simulink model "PMSM_traditional"  (R2014b)
settings: Solver=ode3  StartTime=0.0  StopTime=0.4  FixedStep=10e-6  RelTol=1e-4
libraries: powerlib x6, simulink x1
settings Model: Creator=ZhuJ  LastModifiedBy=Lei
settings SolverCC: SolverResetMethod=Robust
settings DataIOCC: SignalLoggingSaveFormat=ModelDataLogs
settings OptimizationCC: ExpressionDepthLimit=2147483647  InitFltsAndDblsToZero=on
settings DebuggingCC: UnderspecifiedInitializationDetection=Classic  MergeDetectMultiDrivingBlocksExec=none  FcnCallInpInsideContextMsg=UseLocalSettings  StateNameClashWarn=warning
settings GRTTargetCC: CombineOutputUpdateFcns=off  GRTInterface=on

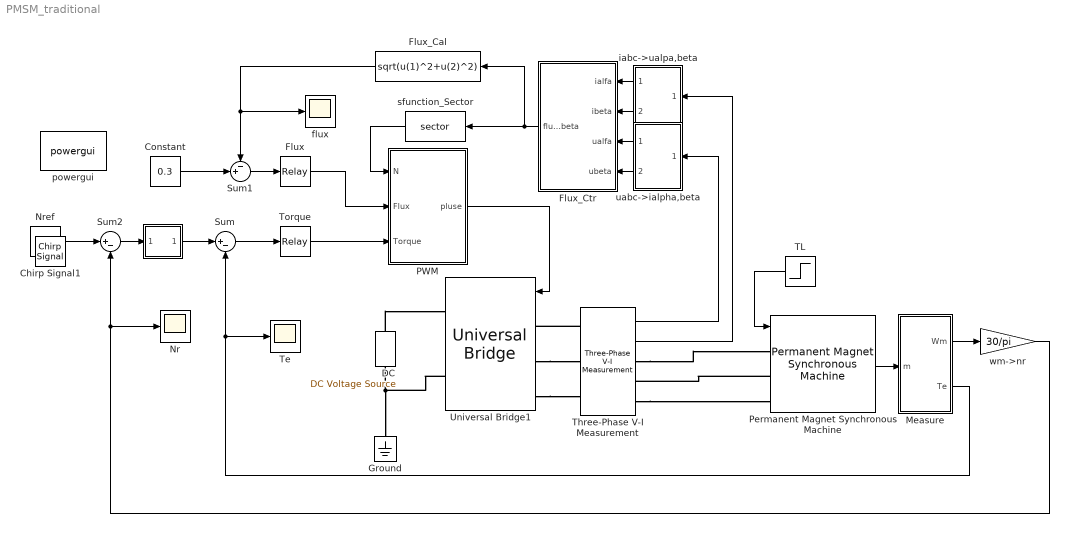
== system PMSM_traditional ==
  "\t" : Subsystem
      mask Display: disp('PI')
  Constant : Constant  Value=0.3
  DC : powerlib/Electrical Sources/DC Voltage Source  Amplitude=311  Measurements=None
  Flux : Relay  OnSwitchValue=0.002  OffSwitchValue=-0.002
  Flux_Cal : Fcn  Expr=sqrt(u(1)^2+u(2)^2)
  Flux_Ctr : Subsystem
  Ground : powerlib/Elements/Ground  LConnTagsString=a
  Measure : Subsystem
  Nr : Scope
      settings: TimeRange=0.3  YMin=595  YMax=620  SaveName=wm  SampleInput=on
  Nref : Constant  Value=600
  PWM : Subsystem
  Permanent Magnet Synchronous Machine : powerlib/Machines/Permanent Magnet Synchronous Machine  NbPhases=3  FluxDistribution=Sinusoidal  RotorType=Salient-pole  MechanicalLoad=Torque Tm  PresetModel=No  ShowDetailedParameters=on  MeasurementBus=off  Resistance=1.2  Inductance=8.5e-3  dqInductances=[8.5e-3,8.5e-3]  La=0.000835  MachineConstant=Flux linkage established by magnets (V.s)  Flux=0.175  VoltageCst=126.966  TorqueCst=1.05  Flat=120  Mechanical=[0.0008 0 4]  PolePairs=4  InitialConditions=[0,0, 0,0]  InitialConditions5ph=[0 0 0 0 0 0]  TsPowergui=0  TsBlock=-1  RefAngle=Aligned with phase A axis (original Park)
  Sum : Sum  Inputs=|+-
  Sum1 : Sum  Inputs=-+|
  Sum2 : Sum  Inputs=|+-
  TL : Step  Time=0.2  After=1.5  SampleTime=0
  Te : Scope
      settings: YMin=-2  SaveName=Te  SampleInput=on
  Three-Phase V-I Measurement : powerlib/Measurements/Three-Phase V-I Measurement  VoltageMeasurement=phase-to-ground  SetLabelV=off  LabelV=Vabc  Vpu=off  VpuLL=off  CurrentMeasurement=yes  SetLabelI=off  LabelI=Iabc  Ipu=off  Pbase=100e6  Vbase=500e3  OutputType=Complex  PhasorSimulation=off  PSBequivalent=0
  Torque : Relay  OnSwitchValue=0.1  OffSwitchValue=-0.1
  Universal Bridge1 : powerlib/Power Electronics/Universal Bridge  Arms=3  SnubberResistance=1e5  SnubberCapacitance=inf  Device=IGBT / Diodes  Ron=1e-3  Lon=0  ForwardVoltages="[  0  0  ]"  ForwardVoltage=0  GTOparameters=[ 10e-6 , 20e-6 ]  IGBTparameters=[ 1e-6 , 2e-6 ]  Measurements=None  Measurements_2=None  converterType=Rectifier
  flux : Scope
      settings: TimeRange=0.3  YMin=-100  YMax=900  SaveName=flux  SampleInput=on
  iabc->ualpa,beta : Subsystem
  powergui : powerlib/powergui  Priority=1  SimulationMode=Continuous  SolverType=Tustin/Backward Euler (TBE)  SampleTime=50e-6  frequency=60  SPID=off  DisableSnubberDevices=off  DisableRonSwitches=off  DisableVfSwitches=off  SwTol=0  DisplayEquations=off  Interpol=off  methode=off  Ts=100  frequencyindice=0  Pbase=100e6  ErrMax=1e-4  Iterations=50  UnitsV=kV  UnitsW=MW  FunctionMessages=off  echomessages=off  HookPort=off  EnableUseOfTLC=off  x0status=blocks  RestoreLinks=warning  ResistiveCurrentMeasurement=off  Frange=[0:2:500]  Ylog=off  Xlog=on  ShowGrid=off  save=off  variable=ZData  structure=0  ZoomFFT=off  StartTime=0.0  cycles=1  DisplayStyle=1  fundamental=60  FreqAxis=off  MaxFrequency=1000  frequencyindicesteady=1  RmsSteady=1  display=off
  sfunction_Sector : S-Function  FunctionName=sector  EnableBusSupport=off
  uabc->ialpha,beta : Subsystem
  wm->nr : Gain  Gain=30/pi
  Chirp Signal1 : simulink/Sources/Chirp Signal  IOType=siggen  f1=0.1  T=100  f2=1
  wires:
  iabc->ualpa,beta/1(ialfa) -> Flux_Ctr/1(ialfa)
  iabc->ualpa,beta/2(ibeta) -> Flux_Ctr/2(ibeta)
  uabc->ialpha,beta/1(ualfa) -> Flux_Ctr/3(ualfa)
  uabc->ialpha,beta/2(ubeta) -> Flux_Ctr/4(ubeta)
  wm->nr/1 -> Nr/1, Sum2/2
  TL/1 -> Permanent Magnet Synchronous Machine/1
  Measure/1(Wm) -> wm->nr/1
  Sum2/1 -> "\t"/1(In1)
  Permanent Magnet Synchronous Machine/1 -> Measure/1(m)
  Flux_Ctr/1(fluxalfa,beta) -> sfunction_Sector/1, Flux_Cal/1
  sfunction_Sector/1 -> PWM/1(N)
  Torque/1 -> PWM/3(Torque)
  "\t"/1(Out1) -> Sum/1
  Sum/1 -> Torque/1
  PWM/1(pluse) -> Universal Bridge1/1
  Measure/2(Te) -> Sum/2, Te/1
  Flux/1 -> PWM/2(Flux)
  Constant/1 -> Sum1/2
  Flux_Cal/1 -> flux/1, Sum1/1
  Sum1/1 -> Flux/1
  Nref/1 -> Sum2/1
  Three-Phase V-I Measurement/1 -> uabc->ialpha,beta/1(uabc)
  Three-Phase V-I Measurement/2 -> iabc->ualpa,beta/1(iabc)
  connections:
  Universal Bridge1/LConn2 -- Three-Phase V-I Measurement/LConn2
  Three-Phase V-I Measurement/LConn1 -- Universal Bridge1/LConn1
  Permanent Magnet Synchronous Machine/LConn2 -- Three-Phase V-I Measurement/RConn2
  Universal Bridge1/LConn3 -- Three-Phase V-I Measurement/LConn3
  Three-Phase V-I Measurement/RConn3 -- Permanent Magnet Synchronous Machine/LConn3
  Three-Phase V-I Measurement/RConn1 -- Permanent Magnet Synchronous Machine/LConn1
  DC/RConn1 -- Universal Bridge1/RConn1
  Universal Bridge1/RConn2 -- Ground/LConn1 -- DC/LConn1

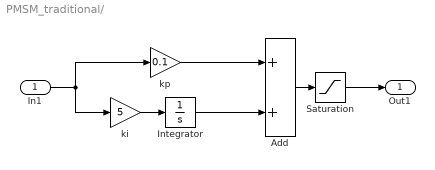
== system PMSM_traditional/	 ==
  In1 : Inport
  Add : Sum
  Integrator : Integrator
  Saturation : Saturate  UpperLimit=5  LowerLimit=-5  LinearizeAsGain=off
  ki : Gain  Gain=5
  kp : Gain  Gain=0.1
  Out1 : Outport
  wires:
  In1/1 -> ki/1, kp/1
  Saturation/1 -> Out1/1
  ki/1 -> Integrator/1
  Add/1 -> Saturation/1
  kp/1 -> Add/1
  Integrator/1 -> Add/2

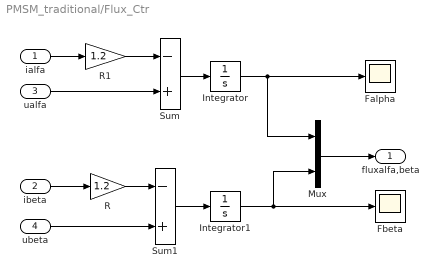
== system PMSM_traditional/Flux_Ctr ==
  ialfa : Inport
  ibeta : Inport  Port=2
  ualfa : Inport  Port=3
  ubeta : Inport  Port=4
  Falpha : Scope
      settings: TimeRange=0.3  YMin=-0.4  YMax=0.4  SaveName=Falpha  SampleInput=on
  Fbeta : Scope
      settings: TimeRange=0.3  YMin=-100  YMax=900  SaveName=Fbeta  SampleInput=on
  Integrator : Integrator
  Integrator1 : Integrator
  Mux : Mux  Inputs=2
  R : Gain  Gain=1.2
  R1 : Gain  Gain=1.2
  Sum : Sum  Inputs=-+
  Sum1 : Sum  Inputs=-+
  fluxalfa,beta : Outport
  wires:
  ualfa/1 -> Sum/2
  ubeta/1 -> Sum1/2
  Sum/1 -> Integrator/1
  Sum1/1 -> Integrator1/1
  Integrator1/1 -> Fbeta/1, Mux/2
  Mux/1 -> fluxalfa,beta/1
  Integrator/1 -> Falpha/1, Mux/1
  ibeta/1 -> R/1
  R/1 -> Sum1/1
  ialfa/1 -> R1/1
  R1/1 -> Sum/1

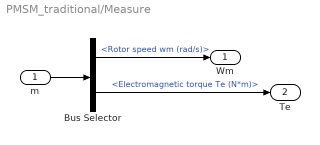
== system PMSM_traditional/Measure ==
  m : Inport
  Bus Selector : BusSelector  OutputSignals=Rotor speed wm (rad/s),Electromagnetic torque Te (N*m)
  Wm : Outport
  Te : Outport  Port=2
  wires:
  Bus Selector/1 -> Wm/1  "<Rotor speed wm (rad/s)>"
  m/1 -> Bus Selector/1
  Bus Selector/2 -> Te/1  "<Electromagnetic torque Te (N*m)>"

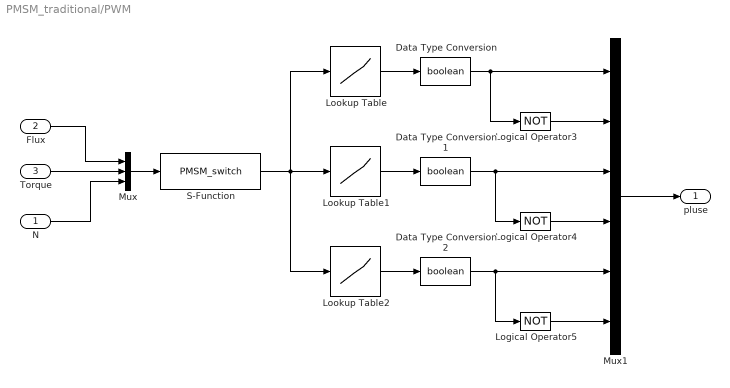
== system PMSM_traditional/PWM ==
  N : Inport
  Flux : Inport  Port=2
  Torque : Inport  Port=3
  Data Type Conversion : DataTypeConversion  OutDataTypeStr=boolean
  Data Type Conversion1 : DataTypeConversion  OutDataTypeStr=boolean
  Data Type Conversion2 : DataTypeConversion  OutDataTypeStr=boolean
  Logical Operator3 : Logic  Operator=NOT  AllPortsSameDT=off  OutDataTypeStr=boolean
  Logical Operator4 : Logic  Operator=NOT  AllPortsSameDT=off  OutDataTypeStr=boolean
  Logical Operator5 : Logic  Operator=NOT  AllPortsSameDT=off  OutDataTypeStr=boolean
  Lookup Table : Lookup  InputValues=[1,2,3,4,5,6]  Table=[1,1,1,0,0,0]
  Lookup Table1 : Lookup  InputValues=[1,2,3,4,5,6]  Table=[1,0,0,1,1,0]
  Lookup Table2 : Lookup  InputValues=[1,2,3,4,5,6]  Table=[0,1,0,1,0,1]
  Mux : Mux  Inputs=3
  Mux1 : Mux  Inputs=6
  S-Function : S-Function  FunctionName=PMSM_switch  EnableBusSupport=off
  pluse : Outport
  wires:
  Torque/1 -> Mux/2
  Flux/1 -> Mux/1
  N/1 -> Mux/3
  Mux/1 -> S-Function/1
  Logical Operator3/1 -> Mux1/2
  Logical Operator4/1 -> Mux1/4
  Logical Operator5/1 -> Mux1/6
  Mux1/1 -> pluse/1
  S-Function/1 -> Lookup Table1/1, Lookup Table/1, Lookup Table2/1
  Lookup Table/1 -> Data Type Conversion/1
  Data Type Conversion/1 -> Mux1/1, Logical Operator3/1
  Lookup Table1/1 -> Data Type Conversion1/1
  Data Type Conversion1/1 -> Mux1/3, Logical Operator4/1
  Lookup Table2/1 -> Data Type Conversion2/1
  Data Type Conversion2/1 -> Mux1/5, Logical Operator5/1

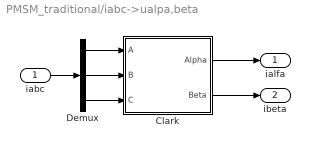
== system PMSM_traditional/iabc->ualpa,beta ==
  iabc : Inport
  Clark : Subsystem
  Demux : Demux  Outputs=3
  ialfa : Outport
  ibeta : Outport  Port=2
  wires:
  iabc/1 -> Demux/1
  Demux/2 -> Clark/2(B)
  Demux/1 -> Clark/1(A)
  Demux/3 -> Clark/3(C)
  Clark/2(Beta) -> ibeta/1
  Clark/1(Alpha) -> ialfa/1

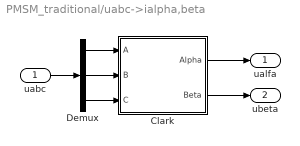
== system PMSM_traditional/uabc->ialpha,beta ==
  uabc : Inport
  Clark : Subsystem
  Demux : Demux  Outputs=3
  ualfa : Outport
  ubeta : Outport  Port=2
  wires:
  uabc/1 -> Demux/1
  Clark/1(Alpha) -> ualfa/1
  Clark/2(Beta) -> ubeta/1
  Demux/2 -> Clark/2(B)
  Demux/1 -> Clark/1(A)
  Demux/3 -> Clark/3(C)

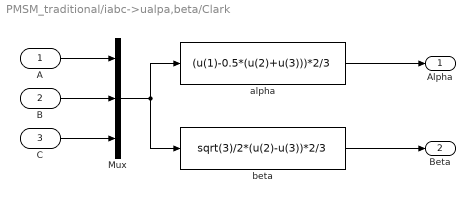
== system PMSM_traditional/iabc->ualpa,beta/Clark ==
  A : Inport
  B : Inport  Port=2
  C : Inport  Port=3
  Mux : Mux  Inputs=3
  alpha : Fcn  Expr=(u(1)-0.5*(u(2)+u(3)))*2/3
  beta : Fcn  Expr=sqrt(3)/2*(u(2)-u(3))*2/3
  Alpha : Outport
  Beta : Outport  Port=2
  wires:
  alpha/1 -> Alpha/1
  B/1 -> Mux/2
  C/1 -> Mux/3
  A/1 -> Mux/1
  Mux/1 -> beta/1, alpha/1
  beta/1 -> Beta/1

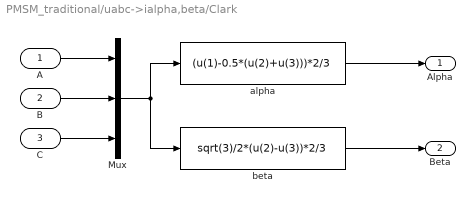
== system PMSM_traditional/uabc->ialpha,beta/Clark ==
  A : Inport
  B : Inport  Port=2
  C : Inport  Port=3
  Mux : Mux  Inputs=3
  alpha : Fcn  Expr=(u(1)-0.5*(u(2)+u(3)))*2/3
  beta : Fcn  Expr=sqrt(3)/2*(u(2)-u(3))*2/3
  Alpha : Outport
  Beta : Outport  Port=2
  wires:
  alpha/1 -> Alpha/1
  B/1 -> Mux/2
  C/1 -> Mux/3
  A/1 -> Mux/1
  Mux/1 -> beta/1, alpha/1
  beta/1 -> Beta/1
